simulink model "AutoEncoderPredictSim"  (R2022a)
settings: Solver=VariableStepAuto  StartTime=0.0  StopTime=labels.Length  RelTol=1e-3
libraries: ReconstructionBlock x1
settings Model: Creator=Alia  LastModifiedBy=Skander
settings SolverCC: AlgebraicLoopSolver=TrustRegion
settings DebuggingCC: UnconnectedInputMsg=warning  UnconnectedOutputMsg=warning  UnconnectedLineMsg=warning  SFMachineParentedDataDiag=warning
settings RTWCC: DLArmComputeVersion=19.05

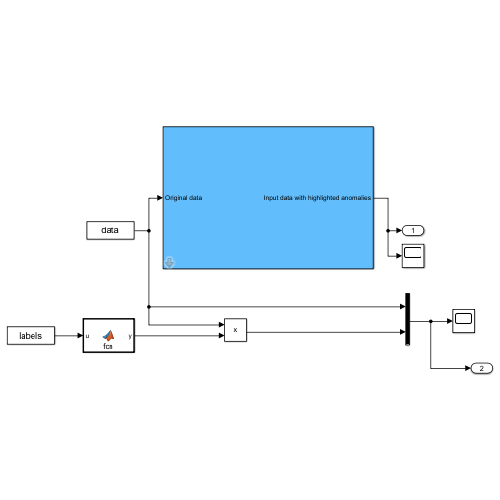
[thumbnail: Simulink's stored preview of the top-level diagram]
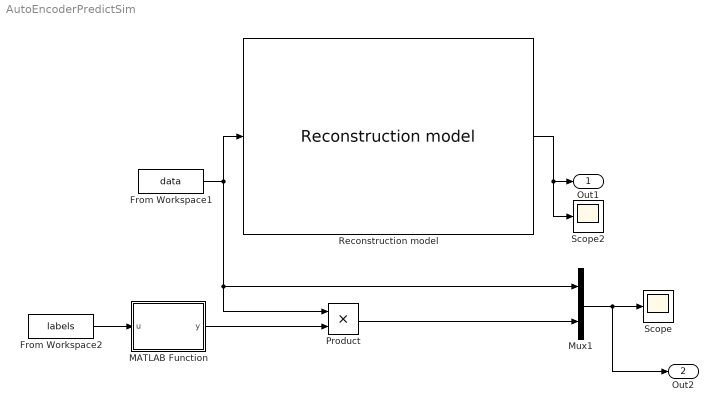
== system AutoEncoderPredictSim ==
  From Workspace1 : FromWorkspace  VariableName=data
  From Workspace2 : FromWorkspace  VariableName=labels
  MATLAB Function : MATLAB Function  TreatAsAtomicUnit=on
  Mux1 : Mux  Inputs=2
  Product : Product
  Reconstruction model : ReconstructionBlock/Reconstruction model
  Scope : Scope
  Scope2 : Scope
  Out1 : Outport
  Out2 : Outport  Port=2
  wires:
  From Workspace2/1 -> MATLAB Function/1(u)
  Product/1 -> Mux1/2
  MATLAB Function/1(y) -> Product/2
  From Workspace1/1 -> Mux1/1, Product/1, Reconstruction model/1
  Mux1/1 -> Out2/1, Scope/1
  Reconstruction model/1 -> Out1/1, Scope2/1

== matlab function AutoEncoderPredictSim/MATLAB Function ==
  data: u input; y output
function y = fcn(u)
y = NaN;
if u == 1
    y = 1;
end
